simulink model "simulink7"  (R2017a)
settings: Solver=VariableStepAuto  StartTime=0.0  StopTime=10  RelTol=1e-3
values from neighbouring files (symbols this model uses):
  C_d = c2d(tf(C), T, 'tustin')    [es7.m]
  G = 1/(s * (s + 1))    [es7.m]
  T = 2 * pi / 1000    (= 0.00628318530718)    [es7.m]
settings Model: Creator=Umberto  LastModifiedBy=Umberto

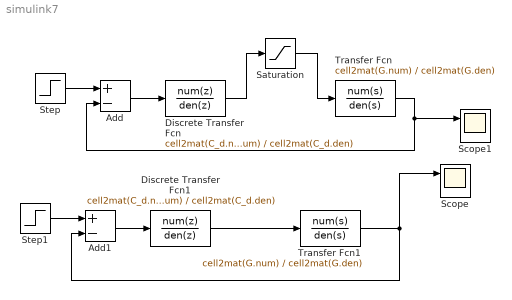
== system simulink7 ==
  Add : Sum  Inputs=+-
  Add1 : Sum  Inputs=+-
  Discrete Transfer Fcn : DiscreteTransferFcn  Numerator=cell2mat(C_d.num)  Denominator=cell2mat(C_d.den)  SampleTime=T
  Discrete Transfer Fcn1 : DiscreteTransferFcn  Numerator=cell2mat(C_d.num)  Denominator=cell2mat(C_d.den)  SampleTime=T
  Saturation : Saturate  UpperLimit=1000  LowerLimit=-1000
  Scope : Scope  NumInputPorts=2
  Scope1 : Scope  NumInputPorts=2
  Step : Step  SampleTime=0
  Step1 : Step  SampleTime=0
  Transfer Fcn : TransferFcn  Numerator=cell2mat(G.num)  Denominator=cell2mat(G.den)
  Transfer Fcn1 : TransferFcn  Numerator=cell2mat(G.num)  Denominator=cell2mat(G.den)
  wires:
  Add/1 -> Discrete Transfer Fcn/1
  Transfer Fcn/1 -> Add/2, Scope1/1
  Step/1 -> Add/1
  Discrete Transfer Fcn/1 -> Saturation/1
  Saturation/1 -> Transfer Fcn/1
  Add1/1 -> Discrete Transfer Fcn1/1
  Step1/1 -> Add1/1
  Transfer Fcn1/1 -> Scope/1, Add1/2
  Discrete Transfer Fcn1/1 -> Transfer Fcn1/1
